simulink model "XPlaneVisualRender"  (R2018a)
settings: Solver=ode23  StartTime=0  StopTime=500  FixedStep=0.001  RelTol=9e-3
model workspace (MAT data in the model file):
  carrera_maxima = Simulink.Parameter
  carrera_maxima.Value = 45
  carrera_maxima.DataType = 'single'
  carrera_maxima.Dimensions = [1 1]
  g_density = 5
libraries: etargetslib x3, dspnetwork x3
settings Model: OrderedModelArguments=off  Creator=Flight Test Lab  LastModifiedBy=Manolo
settings SolverCC: MaxOrder=4  AutoInsertRateTranBlk=on
settings DataIOCC: SaveFormat=StructureWithTime  SaveOutput=off  SignalLogging=off  DSMLogging=off  SaveTime=off
settings OptimizationCC: BlockReduction=off  DefaultUnderspecifiedDataType=single  OptimizeBlockIOStorage=off  BufferReuse=off  GlobalBufferReuse=off  ExpressionFolding=off  LocalBlockOutputs=off  LifeSpan=inf  OptimizeDataStoreBuffers=off  BusAssignmentInplaceUpdate=off
settings DebuggingCC: SFExecutionAtInitializationDiag=none
settings HardwareCC: ProdBitPerSizeT=32  ProdBitPerPtrDiffT=32  ProdWordSize=32  ProdHWDeviceType=Specified
settings RTWCC: Description=Generic Real-Time Target  TargetLang=C++  RTWCompilerOptimization=on
settings CodeAppCC: MaxIdLength=95  StateflowObjectComments=on
settings GRTTargetCC: TargetLangStandard=C++03 (ISO)  MultiInstanceERTCode=on  CodeInterfacePackaging=C++ class

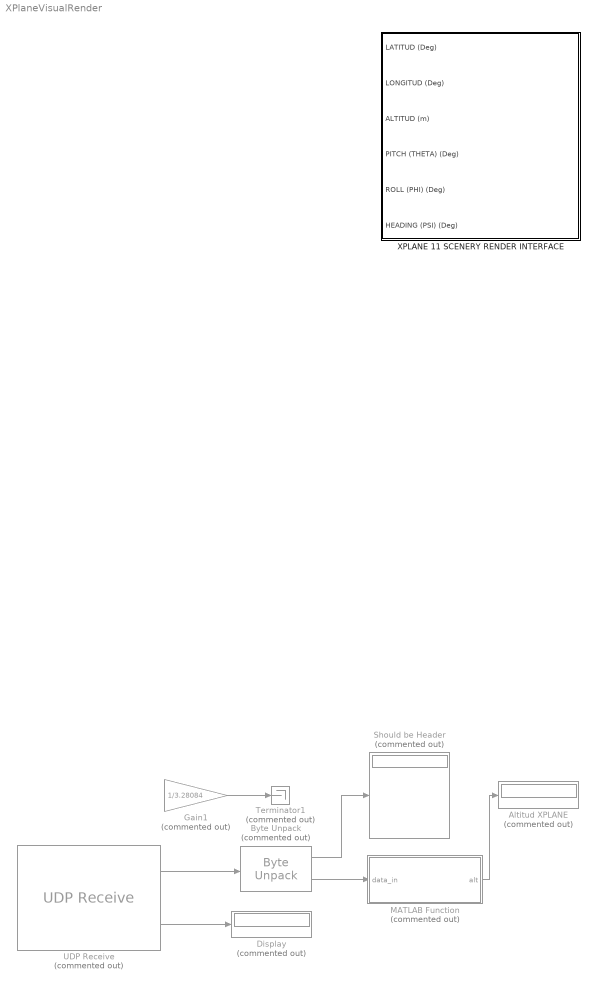
== system XPlaneVisualRender ==
  " XPLANE 11 SCENERY RENDER INTERFACE" : Subsystem  mask{recvport_xplane=49010, sendport_xplane=49000, sendport_dyn=19750, ipxplane='127.0.0.1', ipdyn='255.255.255.255'}
      mask prompts: recvport_xplane "Recepción de datos X-Plane"; sendport_xplane "Envío de datos a X-Plane"; sendport_dyn "Envío de datos a Dynamics"; ipxplane "IP de X-Plane"; ipdyn "IP de Dynamics"
      mask DialogControl ParameterGroupVar Prompt: Puertos
      mask DialogControl Container3 Prompt: IP
  Altitud XPLANE : Display  Commented=on
  Byte Unpack : etargetslib/Byte Unpack  Commented=on  dimensions={5,[1,9]}  datatypes={'uint8','single'}  byteAlign=1
  Display : Display  Commented=on
  Gain1 : Gain  Commented=on  Gain=1/3.28084
  MATLAB Function : MATLAB Function  Commented=on  TreatAsAtomicUnit=on
  Should be Header : Display  Commented=on
  Terminator1 : Terminator  Commented=on
  UDP Receive : dspnetwork/UDP Receive  Commented=on  localURL='0.0.0.0'  localPort=49014  remoteURL='0.0.0.0'  remotePort=-1  recvBufferSize=8192  dims=41  signalDatatype=uint8  isVarSize=off  showBlockingTime=off  blockingTime=0  sampletime=inf  blockPlatform=[]
  wires:
  UDP Receive/2 -> Display/1
  Byte Unpack/1 -> Should be Header/1
  UDP Receive/1 -> Byte Unpack/1
  Byte Unpack/2 -> MATLAB Function/1(data_in)
  MATLAB Function/1(alt) -> Altitud XPLANE/1
  Gain1/1 -> Terminator1/1

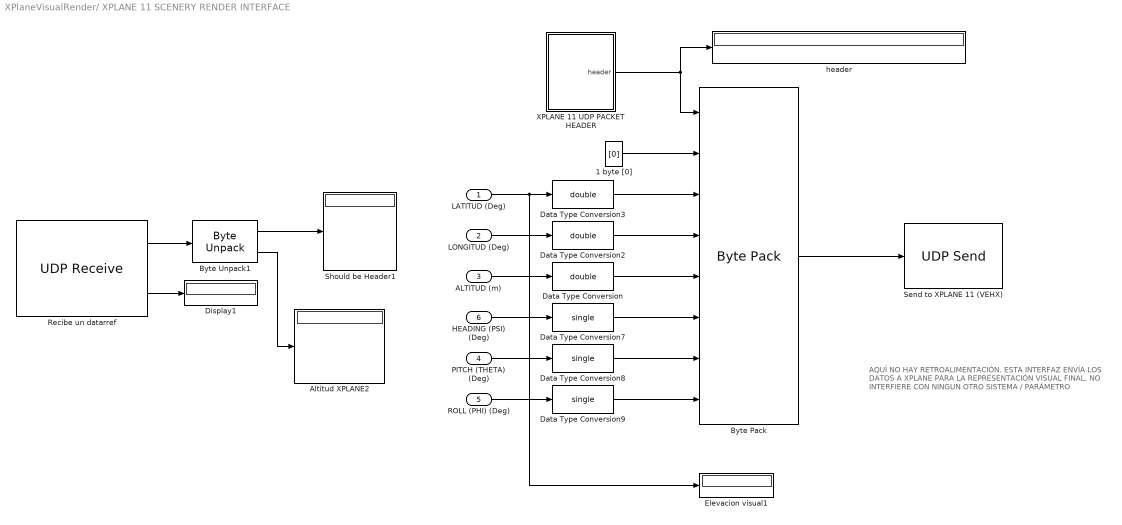
== system XPlaneVisualRender/ XPLANE 11 SCENERY RENDER INTERFACE ==
  note: AQUÍ NO HAY RETROALIMENTACIÓN. ESTA INTERFAZ ENVÍA LOS DATOS
      | A XPLANE PARA LA REPRESENTACIÓN VISUAL FINAL, NO INTERFIERE CON
      | NINGUN OTRO SISTEMA / PARÁMETRO
  LATITUD (Deg) : Inport
  LONGITUD (Deg) : Inport  Port=2
  ALTITUD (m) : Inport  Port=3
  PITCH (THETA) (Deg) : Inport  Port=4
  ROLL (PHI) (Deg) : Inport  Port=5
  HEADING (PSI) (Deg) : Inport  Port=6
  1 byte [0] : Constant  Value=[0]  OutDataTypeStr=single
  Altitud XPLANE2 : Display
      settings: Decimation=5
  Byte Pack : etargetslib/Byte Pack  datatypes={'uint8','single','double','double','double','single','single','single'}  byteAlign=1
  Byte Unpack1 : etargetslib/Byte Unpack  dimensions={5,1}  datatypes={'uint8','single'}  byteAlign=1
  Data Type Conversion : DataTypeConversion  OutDataTypeStr=double
  Data Type Conversion2 : DataTypeConversion  OutDataTypeStr=double
  Data Type Conversion3 : DataTypeConversion  OutDataTypeStr=double
  Data Type Conversion7 : DataTypeConversion  OutDataTypeStr=single
  Data Type Conversion8 : DataTypeConversion  OutDataTypeStr=single
  Data Type Conversion9 : DataTypeConversion  OutDataTypeStr=single
  Display1 : Display
  Elevacion visual1 : Display
  Recibe un datarref : dspnetwork/UDP Receive  localURL='0.0.0.0'  localPort=recvport_xplane  remoteURL=ipxplane  remotePort=-1  recvBufferSize=8192  dims=9  signalDatatype=uint8  isVarSize=off  showBlockingTime=off  blockingTime=0  sampletime=-1  blockPlatform=[]
  Send to XPLANE 11 (VEHX) : dspnetwork/UDP Send  remoteURL=ipxplane  remotePort=sendport_xplane  localURL='0.0.0.0'  localPortSource=Automatically determine  localPort=-1  sampletime=-1  blockPlatform=[]  separateLengthPort=0
  Should be Header1 : Display
  XPLANE 11 UDP PACKET HEADER : MATLAB Function  TreatAsAtomicUnit=on
  header : Display
  wires:
  XPLANE 11 UDP PACKET HEADER/1(header) -> header/1, Byte Pack/1
  Data Type Conversion8/1 -> Byte Pack/7
  1 byte [0]/1 -> Byte Pack/2
  Data Type Conversion9/1 -> Byte Pack/8
  Data Type Conversion/1 -> Byte Pack/5
  Data Type Conversion2/1 -> Byte Pack/4
  Data Type Conversion3/1 -> Byte Pack/3
  Data Type Conversion7/1 -> Byte Pack/6
  HEADING (PSI) (Deg)/1 -> Data Type Conversion7/1
  Byte Pack/1 -> Send to XPLANE 11 (VEHX)/1
  ALTITUD (m)/1 -> Data Type Conversion/1
  LONGITUD (Deg)/1 -> Data Type Conversion2/1
  ROLL (PHI) (Deg)/1 -> Data Type Conversion9/1
  LATITUD (Deg)/1 -> Elevacion visual1/1, Data Type Conversion3/1
  PITCH (THETA) (Deg)/1 -> Data Type Conversion8/1
  Recibe un datarref/1 -> Byte Unpack1/1
  Recibe un datarref/2 -> Display1/1
  Byte Unpack1/1 -> Should be Header1/1
  Byte Unpack1/2 -> Altitud XPLANE2/1

== matlab function XPlaneVisualRender/ XPLANE 11 SCENERY RENDER INTERFACE/XPLANE 11 UDP PACKET HEADER ==
  data: header output uint8
function header  = fcn 
header =[uint8(86) uint8(69) uint8(72) uint8(88) uint8(48)];

 %Surface_header = typecast(uint8([uint8(8) uint8(0) uint8(0) uint8(0)]),'single')
%surfaces_control_cmd = [0 dat_lat dat_lon dat_ele veh_psi_true veh_the veh_phi];
%Throttle_header = typecast(uint8([uint8(25) uint8(0) uint8(0) uint8(0)]),'single');
%throttle_cmd = [3.503246160812043e-44 throttle No_Comand No_Comand No_Comand No_Comand No_Comand No_Comand No_Comand];
end

== matlab function XPlaneVisualRender/MATLAB Function ==
  data: data_in input; alt output
function alt  = decoder(data_in)
 alt = data_in(1,4);

end
